simulink model "W04_4_inner_loop"  (R2024b)
settings: Solver=FixedStepDiscrete  StartTime=0.0  StopTime=inf  FixedStep=0.05  RelTol=1e-3
values from neighbouring files (symbols this model uses):
  animate = 1    [W04_setup.m]
  Kd_psi = -400    [W04_setup.m]
  Ki_psi = 0    [W04_setup.m]
  Kp_psi = 800    [W04_setup.m]
  N_max = 500    [W04_setup.m]
  psi_ref_deg = 45    [W04_setup.m]
  use_ssa = 1    [W04_setup.m]
undefined symbols (not defined in the file or in its folder): DiscIntNeverNeededParam
libraries: ros2lib x5, slpidlib x1
settings Model: Creator=admin  LastModifiedBy=admin

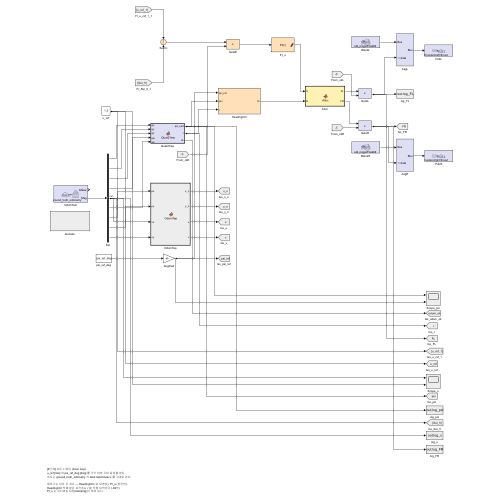
[thumbnail: Simulink's stored preview of the top-level diagram]
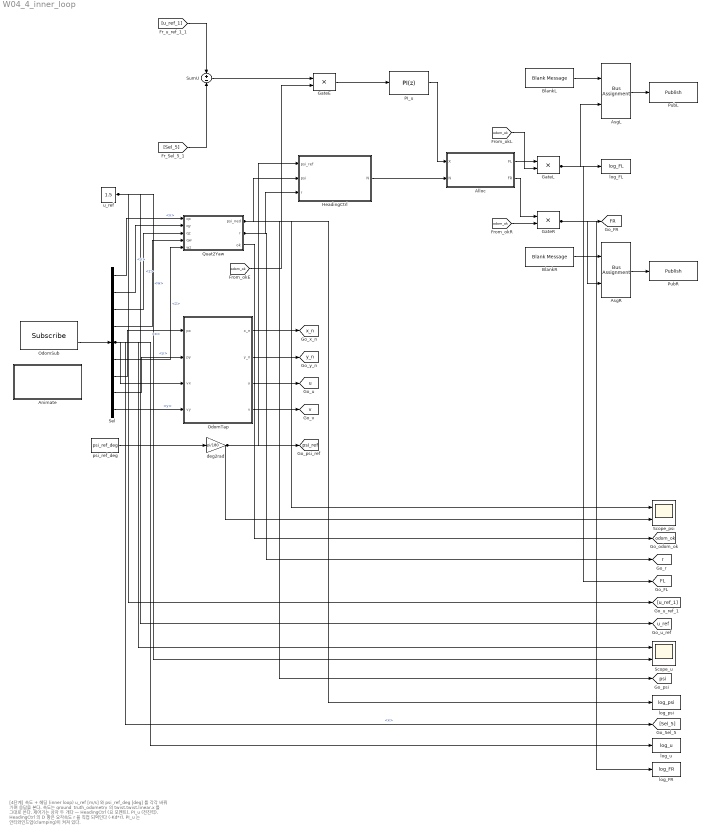
== system W04_4_inner_loop ==
  note: [4단계] 속도 + 헤딩 (inner loop)
      | u_ref [m/s] 와 psi_ref_deg [deg] 를 각각 바꿔 가며 응답을 본다.
      | 속도는 ground_truth_odometry 의 twist.twist.linear.x 를 그대로 쓴다.
      |
      | 제어기는 상자 두 개다 — HeadingCtrl (요 모멘트), PI_u (전진력).
      | HeadingCtrl 의 D 항은 요각속도 r 을 직접 되먹인다 (-Kd*r).
      | PI_u 는 안티와인드업(clamping)이 켜져 있다.
  Alloc : MATLAB Function  TreatAsAtomicUnit=on
  Animate : Subsystem
  AsgL : BusAssignment  AssignedSignals=data
  AsgR : BusAssignment  AssignedSignals=data
  BlankL : ros2lib/Blank Message  messageClass=Message  entityType=std_msgs/Float64  messageType=std_msgs/Float64  SampleTime=0.05
  BlankR : ros2lib/Blank Message  messageClass=Message  entityType=std_msgs/Float64  messageType=std_msgs/Float64  SampleTime=0.05
  GateE : Product
  GateL : Product
  GateR : Product
  HeadingCtrl : Subsystem
  OdomSub : ros2lib/Subscribe  topicSource=Specify your own  topic=/wamv/sensors/position/ground_truth_odometry  messageType=nav_msgs/Odometry  sampleTime=0.05  QOSHistory=Keep last  QOSDepth=1  QOSReliability=Reliable  QOSDurability=Volatile  QOSDeadline=Inf  QOSLifespan=Inf  QOSLiveliness=Automatic  QOSLeaseDuration=Inf  QOSAvoidROSNamespaceConventions=off
  OdomTap : MATLAB Function  TreatAsAtomicUnit=on
  PI_u : slpidlib/PID Controller  Controller=PI  Form=Parallel  TimeDomain=Discrete-time  UseExternalTs=off  SampleTime=0.05  IntegratorMethod=Forward Euler  FilterMethod=Forward Euler  ControllerParametersSource=internal  P=300  I=40  UseKiTs=off  D=0  UseExternalDerivativeSource=off  N=100  UseFilter=on  TunerSelectOption=Transfer Function Based (PID Tuner App)  InitialConditionSource=internal  InitialConditionForIntegrator=0  InitialConditionForFilter=0  DifferentiatorICPrevScaledInput=0  ExternalReset=none  TrackingMode=off  Kt=1  LimitOutput=on  SatLimitsSource=internal  UpperSaturationLimit=500  LowerSaturationLimit=-500  LinearizeAsGain=off  AntiWindupMode=clamping  Kb=1  LimitIntegrator=off  UpperIntegratorSaturationLimit=inf  LowerIntegratorSaturationLimit=-inf  POutMin=[]  POutMax=[]  IOutMin=[]  IOutMax=[]  DOutMin=[]  DOutMax=[]  NOutMin=[]  NOutMax=[]  SumOutMin=[]  SumOutMax=[]  SaturationOutMin=[]  SaturationOutMax=[]  PParamMin=[]  PParamMax=[]  IParamMin=[]  IParamMax=[]  DParamMin=[]  DParamMax=[]  NParamMin=[]  NParamMax=[]  KbParamMin=[]  KbParamMax=[]  KtParamMin=[]  KtParamMax=[]  KbOutMin=[]  KbOutMax=[]  KtOutMin=[]  KtOutMax=[]  IntegratorOutMin=[]  IntegratorOutMax=[]  FilterOutMin=[]  FilterOutMax=[]  SumI1OutMin=[]  SumI1OutMax=[]  SumI2OutMin=[]  SumI2OutMax=[]  SumI3OutMin=[]  SumI3OutMax=[]  SumI4OutMin=[]  SumI4OutMax=[]  SumDOutMin=[]  SumDOutMax=[]  DifferentiatorOutMin=[]  DifferentiatorOutMax=[]  FilterDiffOutCoefMin=[]  FilterDiffOutCoefMax=[]  ReciprocalOutMin=[]  ReciprocalOutMax=[]  SumDenOutMin=[]  SumDenOutMax=[]  SumNumOutMin=[]  SumNumOutMax=[]  DivideOutMin=[]  DivideOutMax=[]  UdiffTsProdOutMin=[]  UdiffTsProdOutMax=[]  NTsProdOutMin=[]  NTsProdOutMax=[]  UintegralTsProdOutMin=[]  UintegralTsProdOutMax=[]  UngainTsProdOutMin=[]  UngainTsProdOutMax=[]  ClampingZeroOutDataTypeStr=Inherit: Inherit via back propagation  ClampingZeroOutMin=[]  ClampingZeroOutMax=[]  FilterDenConstantOutDataTypeStr=Inherit: Inherit via back propagation  FilterDenConstantOutMin=[]  FilterDenConstantOutMax=[]  PCopyOutDataTypeStr=Inherit: Inherit via back propagation  PCopyOutMin=[]  PCopyOutMax=[]  NCopyOutDataTypeStr=Inherit: Inherit via back propagation  NCopyOutMin=[]  NCopyOutMax=[]  IntegratorContinuousStateAttributes=''  IntegratorStateMustResolveToSignalObject=off  IntegratorRTWStateStorageClass=Auto  FilterContinuousStateAttributes=''  FilterStateMustResolveToSignalObject=off  FilterRTWStateStorageClass=Auto  ParallelPVariant=InternalParameters  IdealPVariant=Disabled  IVariant=InternalParameters  DVariant=Disabled  IntegratorVariant=Discrete  SatVariant=Enabled  AWVariant=DiscClampingParallel  PCopyVariant=Disabled  TRVariant=Disabled  FdbkBlocksVariant=Forward  IdealPFdbkVariant=Disabled  SatFdbkVariant=Disabled  DerivativeFilterVariant=Disabled  NVariant=Disabled  NCopyVariant=Disabled_SignalSpec  FilterICVariant=Disabled  IntegratorICVariant=InternalICs  ExternalResetVariant=Disabled  TRSumVariant=Passthrough  SumFdbkVariant=Disabled  SumVariant=Sum_PI  TsampFilterVariant=InternalTs  TsampNgainVariant=Passthrough  TsampIntegralVariant=Disabled_SignalSpec  ExternalSaturationOutDataTypeStr=Inherit: Same as second input  DerivativeSourceVariant=Disabled  PreIntVariant=InternalPreInt
      settings: LibrarySourceBlock=simulink/Discrete/Discrete PID Controller
  PubL : ros2lib/Publish  topicSource=Specify your own  topic=/wamv/thrusters/left/thrust  messageType=std_msgs/Float64  QOSHistory=Keep last  QOSDepth=1  QOSReliability=Reliable  QOSDurability=Volatile  QOSDeadline=Inf  QOSLifespan=Inf  QOSLiveliness=Automatic  QOSLeaseDuration=Inf  QOSAvoidROSNamespaceConventions=off
  PubR : ros2lib/Publish  topicSource=Specify your own  topic=/wamv/thrusters/right/thrust  messageType=std_msgs/Float64  QOSHistory=Keep last  QOSDepth=1  QOSReliability=Reliable  QOSDurability=Volatile  QOSDeadline=Inf  QOSLifespan=Inf  QOSLiveliness=Automatic  QOSLeaseDuration=Inf  QOSAvoidROSNamespaceConventions=off
  Quat2Yaw : MATLAB Function  TreatAsAtomicUnit=on
  Scope_psi : Scope  NumInputPorts=2
  Scope_u : Scope  NumInputPorts=2
  Sel : BusSelector  OutputSignals=pose.pose.orientation.x,pose.pose.orientation.y,pose.pose.orientation.z,pose.pose.orientation.w,twist.twist.linear.x,twist.twist.angular.z,pose.pose.position.x,pose.pose.position.y,twist.twist.linear.y
  SumU : Sum  Inputs=+-
  deg2rad : Gain  Gain=pi/180
  log_FL : ToWorkspace  VariableName=log_FL  SaveFormat=Timeseries  SampleTime=0.05
  log_FR : ToWorkspace  VariableName=log_FR  SaveFormat=Timeseries  SampleTime=0.05
  log_psi : ToWorkspace  VariableName=log_psi  SaveFormat=Timeseries  SampleTime=0.05
  log_u : ToWorkspace  VariableName=log_u  SaveFormat=Timeseries  SampleTime=0.05
  psi_ref_deg : Constant  Value=psi_ref_deg
  u_ref : Constant  Value=1.5
  tag scope: FL=global, FR=global, odom_ok=global, psi=global, psi_ref=global, r=global, u=global, u_ref=global, v=global, x_n=global, y_n=global
  wires:
  GateR/1 -> AsgR/2, [FR], log_FR/1
  Sel/5 -> OdomTap/3(vx), [Sel_5], Scope_u/1, log_u/1  "<x>"
  Quat2Yaw/1(psi_ned) -> HeadingCtrl/2(psi), [psi], Scope_psi/1, log_psi/1
  SumU/1 -> GateE/1
  OdomSub/2 -> Sel/1
  Sel/4 -> Quat2Yaw/4(qw)  "<w>"
  [odom_ok] -> GateR/2
  Sel/1 -> Quat2Yaw/1(qx)  "<x>"
  PI_u/1 -> Alloc/1(X)
  Sel/2 -> Quat2Yaw/2(qy)  "<y>"
  Sel/3 -> Quat2Yaw/3(qz)  "<z>"
  Sel/6 -> Quat2Yaw/5(wz)  "<z>"
  Sel/7 -> OdomTap/1(px)  "<x>"
  Sel/8 -> OdomTap/2(py)  "<y>"
  GateL/1 -> log_FL/1, AsgL/2, [FL]
  Sel/9 -> OdomTap/4(vy)  "<y>"
  psi_ref_deg/1 -> deg2rad/1
  Quat2Yaw/2(r) -> HeadingCtrl/3(r), [r]
  [odom_ok] -> GateE/2
  OdomTap/1(x_n) -> [x_n]
  OdomTap/2(y_n) -> [y_n]
  OdomTap/3(u) -> [u]
  OdomTap/4(v) -> [v]
  deg2rad/1 -> HeadingCtrl/1(psi_ref), [psi_ref], Scope_psi/2
  GateE/1 -> PI_u/1
  HeadingCtrl/1(N) -> Alloc/2(N)
  [odom_ok] -> GateL/2
  BlankL/1 -> AsgL/1
  Alloc/1(FL) -> GateL/1
  Alloc/2(FR) -> GateR/1
  BlankR/1 -> AsgR/1
  AsgL/1 -> PubL/1
  AsgR/1 -> PubR/1
  [Sel_5] -> SumU/2
  Quat2Yaw/3(ok) -> [odom_ok]
  u_ref/1 -> [u_ref_1], [u_ref], Scope_u/2
  [u_ref_1] -> SumU/1

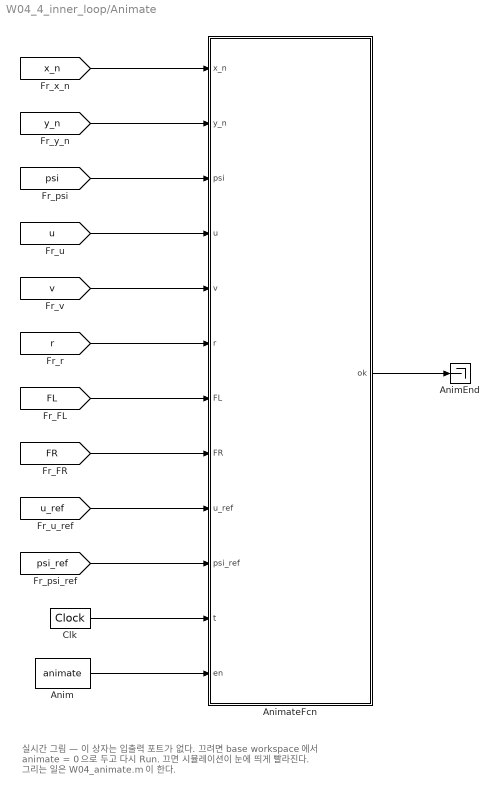
== system W04_4_inner_loop/Animate ==
  note: 실시간 그림 — 이 상자는 입출력 포트가 없다.
      | 끄려면 base workspace 에서  animate = 0  으로 두고 다시 Run.
      | 끄면 시뮬레이션이 눈에 띄게 빨라진다.
      | 그리는 일은 W04_animate.m 이 한다.
  Anim : Constant  Value=animate
  AnimEnd : Terminator
  AnimateFcn : MATLAB Function  TreatAsAtomicUnit=on
  Clk : DigitalClock  SampleTime=0.05
  wires:
  [x_n] -> AnimateFcn/1(x_n)
  [y_n] -> AnimateFcn/2(y_n)
  [psi] -> AnimateFcn/3(psi)
  [u] -> AnimateFcn/4(u)
  [v] -> AnimateFcn/5(v)
  [r] -> AnimateFcn/6(r)
  [FL] -> AnimateFcn/7(FL)
  [FR] -> AnimateFcn/8(FR)
  [u_ref] -> AnimateFcn/9(u_ref)
  [psi_ref] -> AnimateFcn/10(psi_ref)
  Clk/1 -> AnimateFcn/11(t)
  Anim/1 -> AnimateFcn/12(en)
  AnimateFcn/1(ok) -> AnimEnd/1

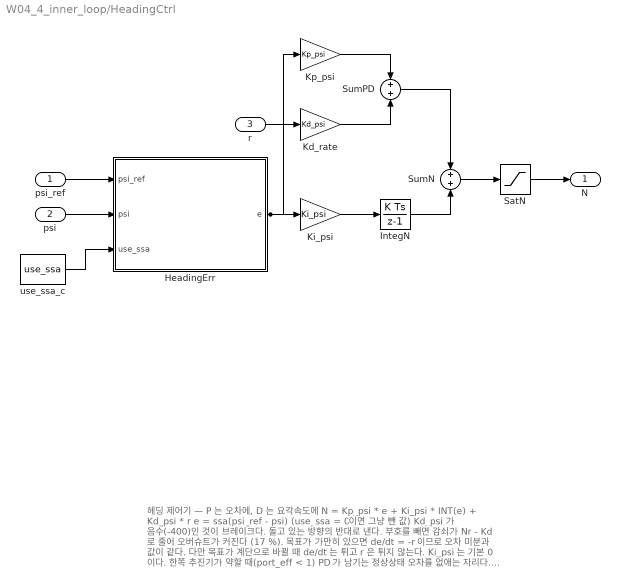
== system W04_4_inner_loop/HeadingCtrl ==
  note: 헤딩 제어기 — P 는 오차에, D 는 요각속도에
      |
      |     N = Kp_psi * e  +  Ki_psi * INT(e)  +  Kd_psi * r
      |     e = ssa(psi_ref - psi)   (use_ssa = 0 이면 그냥 뺀 값)
      |
      | Kd_psi 가 음수(-400)인 것이 브레이크다. 돌고 있는 방향의 반대로 낸다.
      | 부호를 빼면 감쇠가 Nr - Kd 로 줄어 오버슈트가 커진다 (17 %).
      |
      | 목표가 가만히 있으면 de/dt = -r 이므로 오차 미분과 값이 같다.
      | 다만 목표가 계단으로 바뀔 때 de/dt 는 튀고 r 은 튀지 않는다.
      |
      | Ki_psi 는 기본 0 이다. 한쪽 추진기가 약할 때(port_eff < 1)
      | PD 가 남기는 정상상태 오차를 없애는 자리다.
      | 적분기에는 +-N_max 포화가 걸려 있다 (clamping 안티와인드업).
      |
      | 값은 전부 W04_setup.m — Kp_psi = 800, Kd_psi = -400.
      | 근거는 4주차 극배치 절과 W04_pole_place.m.
  psi_ref : Inport
  psi : Inport  Port=2
  r : Inport  Port=3
  HeadingErr : MATLAB Function  TreatAsAtomicUnit=on
  IntegN : DiscreteIntegrator  SampleTime=0.05  LimitOutput=on  UpperSaturationLimit=N_max  LowerSaturationLimit=-N_max  ICPrevOutput=DiscIntNeverNeededParam  ICPrevScaledInput=DiscIntNeverNeededParam
  Kd_rate : Gain  Gain=Kd_psi
  Ki_psi : Gain  Gain=Ki_psi
  Kp_psi : Gain  Gain=Kp_psi
  SatN : Saturate  UpperLimit=N_max  LowerLimit=-N_max
  SumN : Sum
  SumPD : Sum
  use_ssa_c : Constant  Value=use_ssa
  N : Outport
  wires:
  psi_ref/1 -> HeadingErr/1(psi_ref)
  psi/1 -> HeadingErr/2(psi)
  Ki_psi/1 -> IntegN/1
  use_ssa_c/1 -> HeadingErr/3(use_ssa)
  Kp_psi/1 -> SumPD/1
  r/1 -> Kd_rate/1
  HeadingErr/1(e) -> Kp_psi/1, Ki_psi/1
  Kd_rate/1 -> SumPD/2
  SumPD/1 -> SumN/1
  IntegN/1 -> SumN/2
  SumN/1 -> SatN/1
  SatN/1 -> N/1

== matlab function W04_4_inner_loop/OdomTap ==
  data: px input; x_n output; py input; vx input; vy input; y_n output; u output; v output
function [x_n, y_n, u, v] = OdomTap(px, py, vx, vy)
%#codegen
% Ground truth odometry -> the numbers the live plot draws.
% Display only: nothing here feeds the controller.
x_n = py;      % ENU y is north
y_n = px;      % ENU x is east
u   =  vx;     % surge is the same in FLU and NED body axes
v   = -vy;     % FLU +y is port, NED +y is starboard

== matlab function W04_4_inner_loop/Quat2Yaw ==
  data: qx input; psi_ned output; qy input; qz input; qw input; wz input; r output; ok output
function [psi_ned, r, ok] = Quat2Yaw(qx, qy, qz, qw, wz)
%#codegen
% ROS quaternion (ENU body) -> NED heading [rad] and yaw rate [rad/s]
yaw_enu = atan2(2*(qw*qz + qx*qy), 1 - 2*(qy*qy + qz*qz));
psi = pi/2 - yaw_enu;
psi_ned = atan2(sin(psi), cos(psi));   % wrap to [-pi, pi]

% psi_ned = pi/2 - yaw_enu  ->  d(psi_ned)/dt = -d(yaw_enu)/dt.
% ENU is z-up and NED is z-down, so the turn direction flips.
r = -wz;

% ok = 0 holds the thrusters at 0 (addFirstMsgGate). Two reasons:
%  1) Before the first odometry arrives the Subscribe block outputs an all-zero bus.
%     A zero quaternion reads as exactly 90 deg.
%  2) Simulink stalls for up to a few wall-clock seconds in its first steps while
%     Gazebo keeps running on the first thrust command. The boat turned 9 to 55 deg
%     before the model resumed (2026-09-24). So wait 1 s (20 samples) after the first
%     valid message, then start the step from a boat that is still at rest.
persistent n
if isempty(n), n = 0; end
valid = qx ~= 0 || qy ~= 0 || qz ~= 0 || qw ~= 0;
if valid, n = n + 1; end
ok = double(valid && n > 20);

== matlab function W04_4_inner_loop/HeadingCtrl/HeadingErr ==
  data: psi_ref input; e output; psi input; use_ssa input
function e = HeadingErr(psi_ref, psi, use_ssa)
%#codegen
% Heading error [rad].
d = psi_ref - psi;
if use_ssa >= 0.5
    % ssa : shortest signed angle, wrapped to (-pi, pi]
    e = atan2(sin(d), cos(d));
else
    % no wrap : 170 deg -> -170 deg becomes -340 deg, not +20 deg
    e = d;
end

== matlab function W04_4_inner_loop/Alloc ==
  data: X input; FL output; N input; FR output
function [FL, FR] = Alloc(X, N)
%#codegen
% Differential thrust allocation for the 2-thruster WAM-V
%   X : surge force  [N]
%   N : yaw moment   [N*m], positive turns to starboard
B_half = 1.027135;      % half distance between thrusters [m]
Fmax   = 250;           % thrust limit per thruster [N]
FL = X/2 + N/(2*B_half);
FR = X/2 - N/(2*B_half);
FL = max(min(FL, Fmax), -Fmax);
FR = max(min(FR, Fmax), -Fmax);

== matlab function W04_4_inner_loop/Animate/AnimateFcn ==
  data: x_n input; y_n input; psi input; u input; ok output; v input; r input; FL input; FR input; u_ref input; psi_ref input; t input; en input
function ok = AnimateFcn(x_n, y_n, psi, u, v, r, FL, FR, u_ref, psi_ref, t, en)
%#codegen
% 실시간 그림. MATLAB Function 블록은 그림을 그리지 못하므로 그리는 함수를
% extrinsic 으로 선언한다 — 코드를 만들지 않고 평범한 MATLAB 을 부른다.
% en = base workspace 의 animate (0 이면 그리지 않는다).
coder.extrinsic('W04_animate');
ok = 1;
if en > 0.5
    W04_animate(x_n, y_n, psi, u, v, r, FL, FR, u_ref, psi_ref, t);
end
